simulink model "foc_fuzzy"  (R2025b)
settings: Solver=VariableStepAuto  StartTime=0.0  StopTime=3  RelTol=1e-3
libraries: slpidlib x2, spsSVPWMGenerator2LevelLib x1, spsdq0toAlphaBetaZeroLib x1, spsPermanentMagnetSynchronousMachineLib x1, spsDCVoltageSourceLib x1, spsThreePhaseVIMeasurementLib x1, spsUniversalBridgeLib x1, fuzblock x1, spsAlphaBetaZerotodq0Lib x1, spsabctoAlphaBetaZeroLib x1, sps_lib x1
settings Model: Creator=DELL  LastModifiedBy=DELL
settings DataIOCC: SaveState=on  SignalLogging=off  DSMLogging=off  ReturnWorkspaceOutputs=off

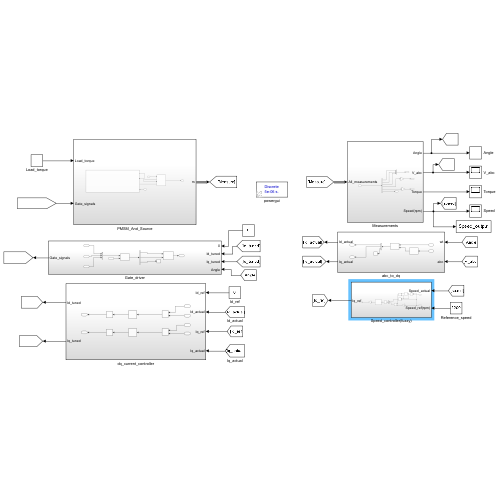
[thumbnail: Simulink's stored preview of the top-level diagram]
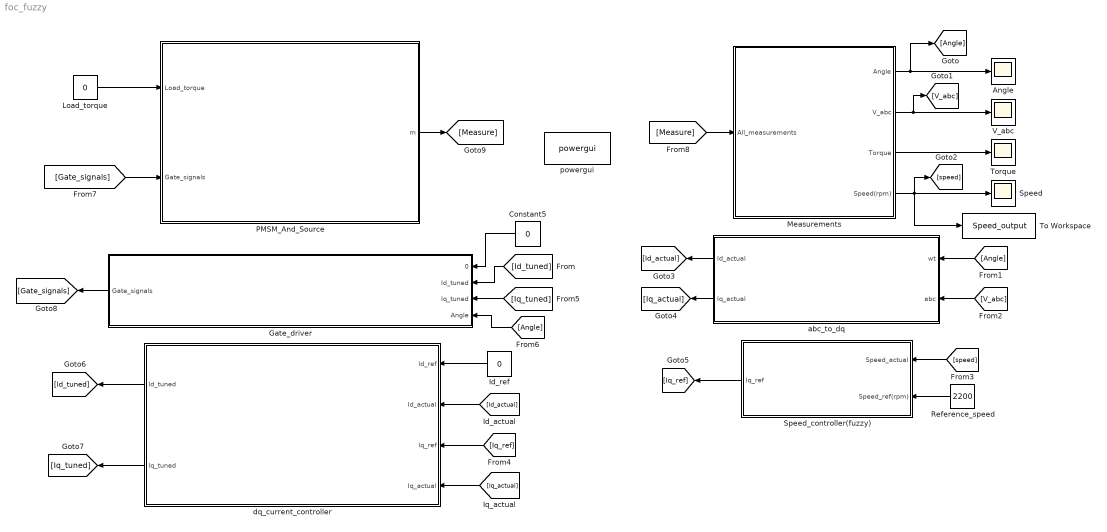
== system foc_fuzzy ==
  Angle : Scope
  Constant5 : Constant  Value=0
  Gate_driver : Subsystem
  Id_ref : Constant  Value=0
  Load_torque : Constant  Value=0
  Measurements : Subsystem
  PMSM_And_Source : Subsystem
  Reference_speed : Constant  Value=2200
  Speed : Scope
      settings: ActiveDisplayYMinimum=-270.85965206876136  ActiveDisplayYMaximum=2437.7368686188529  DataLoggingVariableName=ScopeData3
  Speed_controller(fuzzy) : Subsystem
      settings: PortSchema="{\"entries\":[{\"content\":{\"sides\":[{\"content\":{\"connectorIds\":[\"Out1\"]},\"type\":\"ConnectorPlacement.EquallySpacedRectSide\",\"uuid\":\"a1cd0f4b-38ea-419f-afc2-39e9bc7b0de2\"},{\"content\":{\"connectorIds\":[\"In1\",\"In2\"],\"side\":\"RIGHT\"},\"type\":\"ConnectorPlacement.EquallySpacedRectSide\",\"uuid\":\"efef469d-788b-4725-983f-524fe539f85d\"},{\"content\":{\"side\":\"TOP\"},\"type\":\"ConnectorPlacement.EquallySpacedRectSide\",\"uuid\":\"0e401ee3-352a-4969-a305-667f2f0ad6e7\"}]},\"type\":\"ConnectorPlacement.EquallySpacedConnector\",\"uuid\":\"94f18982-1906-49e5-aac5-92abf80968c3\"}],\"packageUris\":[\"http://schema.mathworks.com/mf0/Connector/R2020b\"],\"version\":\"1.0\"}"
  To Workspace : ToWorkspace  VariableName=Speed_output  SampleTime=-1
  Torque : Scope
      settings: DataLoggingVariableName=ScopeData2
  V_abc : Scope
  abc_to_dq : Subsystem
      settings: PortSchema="{\"entries\":[{\"content\":{\"sides\":[{\"content\":{\"connectorIds\":[\"Out1\",\"Out2\"]},\"type\":\"ConnectorPlacement.EquallySpacedRectSide\",\"uuid\":\"7ac698e7-d270-4bd0-8d73-3bcbd5b3bd28\"},{\"content\":{\"connectorIds\":[\"In1\",\"In2\"],\"side\":\"RIGHT\"},\"type\":\"ConnectorPlacement.EquallySpacedRectSide\",\"uuid\":\"e26e1610-01d9-4f07-bf5c-31b1329ae751\"},{\"content\":{\"side\":\"TOP\"},\"type\":\"ConnectorPlacement.EquallySpacedRectSide\",\"uuid\":\"585fc40b-a7d1-43b5-ab48-882fc2ec0db2\"}]},\"type\":\"ConnectorPlacement.EquallySpacedConnector\",\"uuid\":\"4680cdbc-79eb-4a7f-9529-209119af11d2\"}],\"packageUris\":[\"http://schema.mathworks.com/mf0/Connector/R2020b\"],\"version\":\"1.0\"}"
  dq_current_controller : Subsystem
      settings: PortSchema="{\"entries\":[{\"content\":{\"sides\":[{\"content\":{\"connectorIds\":[\"Out1\",\"Out2\"]},\"type\":\"ConnectorPlacement.EquallySpacedRectSide\",\"uuid\":\"85abe6a4-f46d-437d-9d29-ea06215c210d\"},{\"content\":{\"connectorIds\":[\"In1\",\"In2\",\"In3\",\"In4\"],\"side\":\"RIGHT\"},\"type\":\"ConnectorPlacement.EquallySpacedRectSide\",\"uuid\":\"dede3f64-84eb-4a1d-a083-0a7c4f3ca0cd\"},{\"content\":{\"side\":\"TOP\"},\"type\":\"ConnectorPlacement.EquallySpacedRectSide\",\"uuid\":\"b0cb4f54-dbd0-4970-9888-3ed028a2486f\"}]},\"type\":\"ConnectorPlacement.EquallySpacedConnector\",\"uuid\":\"91272fe0-95ae-4ab4-bc55-5dc81673f5f4\"}],\"packageUris\":[\"http://schema.mathworks.com/mf0/Connector/R2020b\"],\"version\":\"1.0\"}"
  powergui : sps_lib/powergui  Priority=1  SimulationMode=Discrete  SampleTime=5e-6  frequency=60  Iterations=50  frequencyindice=0  Pbase=100e6  ErrMax=1e-4  UnitsV=kV  UnitsW=MW  buscounter=0  FunctionMessages=off  echomessages=off  EnableUseOfTLC=off  CurrentSourceSwitches=off  DisableSnubberDevices=off  DisableRonSwitches=off  DisableVfSwitches=off  DisplayEquations=off  AutomaticDiscreteSolvers=off  SolverType=Tustin/Backward Euler (TBE)  Interpol=off  ExternalGateDelay=off  methode=off  Ts=100  x0status=blocks  SPID=on  SwTol=0  HookPort=off  NonlinearTolerance=1e-4  nMaxIteration=100  ContinueOnMaxIteration=off  RestoreLinks=warning  ResistiveCurrentMeasurement=off  Frange=[0:2:500]  Ylog=off  Xlog=on  ShowGrid=off  save=off  variable=ZData  structure=0  ZoomFFT=off  StartTime=0.0  cycles=1  DisplayStyle=1  fundamental=60  FreqAxis=off  MaxFrequency=1000  frequencyindicesteady=1  RmsSteady=1  display=off
  wires:
  Measurements/1(Angle) -> [Angle], Angle/1
  Measurements/2(V_abc) -> V_abc/1, [V_abc]
  Measurements/4(Speed(rpm)) -> To Workspace/1, Speed/1, [speed]
  Measurements/3(Torque) -> Torque/1
  [speed] -> Speed_controller(fuzzy)/1(Speed_actual)
  [Angle] -> abc_to_dq/1(wt)
  [V_abc] -> abc_to_dq/2(abc)
  abc_to_dq/1(Id_actual) -> [Id_actual]
  abc_to_dq/2(Iq_actual) -> [Iq_actual]
  Speed_controller(fuzzy)/1(Iq_ref) -> [Iq_ref]
  Id_ref/1 -> dq_current_controller/1(Id_ref)
  [Id_actual] -> dq_current_controller/2(Id_actual)
  [Iq_ref] -> dq_current_controller/3(Iq_ref)
  [Iq_actual] -> dq_current_controller/4(Iq_actual)
  Constant5/1 -> Gate_driver/1(0)
  dq_current_controller/2(Iq_tuned) -> [Iq_tuned]
  dq_current_controller/1(Id_tuned) -> [Id_tuned]
  [Id_tuned] -> Gate_driver/2(Id_tuned)
  [Iq_tuned] -> Gate_driver/3(Iq_tuned)
  [Angle] -> Gate_driver/4(Angle)
  Gate_driver/1(Gate_signals) -> [Gate_signals]
  [Gate_signals] -> PMSM_And_Source/2(Gate_signals)
  PMSM_And_Source/1(m) -> [Measure]
  [Measure] -> Measurements/1(All_measurements)
  Load_torque/1 -> PMSM_And_Source/1(Load_torque)
  Reference_speed/1 -> Speed_controller(fuzzy)/2(Speed_ref(rpm))

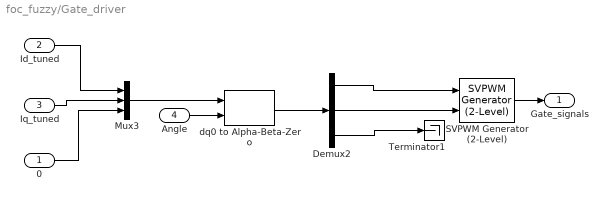
== system foc_fuzzy/Gate_driver ==
  0 : Inport
  Id_tuned : Inport  Port=2
  Iq_tuned : Inport  Port=3
  Angle : Inport  Port=4
  Demux2 : Demux  Outputs=3
  Mux3 : Mux  Inputs=3
  SVPWM Generator (2-Level) : spsSVPWMGenerator2LevelLib/SVPWM Generator (2-Level)  InputType=alpha-beta components  SwitchingPattern=Pattern #1  Fc=5000  ParUref=[0.8 -30 50]  Ts=0
  Terminator1 : Terminator
  dq0 to Alpha-Beta-Zero : spsdq0toAlphaBetaZeroLib/dq0 to Alpha-Beta-Zero  Alignment=90 degrees behind phase A axis
  Gate_signals : Outport
  wires:
  SVPWM Generator (2-Level)/1 -> Gate_signals/1
  Demux2/1 -> SVPWM Generator (2-Level)/1
  Demux2/2 -> SVPWM Generator (2-Level)/2
  Angle/1 -> dq0 to Alpha-Beta-Zero/2
  Demux2/3 -> Terminator1/1
  dq0 to Alpha-Beta-Zero/1 -> Demux2/1
  Mux3/1 -> dq0 to Alpha-Beta-Zero/1
  0/1 -> Mux3/3
  Id_tuned/1 -> Mux3/1
  Iq_tuned/1 -> Mux3/2

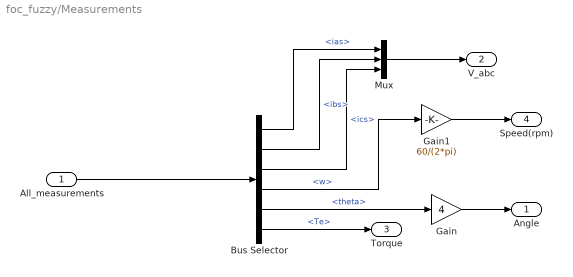
== system foc_fuzzy/Measurements ==
  All_measurements : Inport
  Bus Selector : BusSelector  OutputSignals=ias,ibs,ics,w,theta,Te
  Gain : Gain  Gain=4
  Gain1 : Gain  Gain=60/(2*pi)
  Mux : Mux  Inputs=3
  Angle : Outport
  V_abc : Outport  Port=2
  Torque : Outport  Port=3  VectorParamsAs1DForOutWhenUnconnected=off
  Speed(rpm) : Outport  Port=4
  wires:
  Mux/1 -> V_abc/1
  Gain1/1 -> Speed(rpm)/1
  Bus Selector/4 -> Gain1/1  "<w>"
  Bus Selector/6 -> Torque/1  "<Te>"
  Bus Selector/5 -> Gain/1  "<theta>"
  Bus Selector/3 -> Mux/3  "<ics>"
  Gain/1 -> Angle/1
  Bus Selector/1 -> Mux/1  "<ias>"
  Bus Selector/2 -> Mux/2  "<ibs>"
  All_measurements/1 -> Bus Selector/1

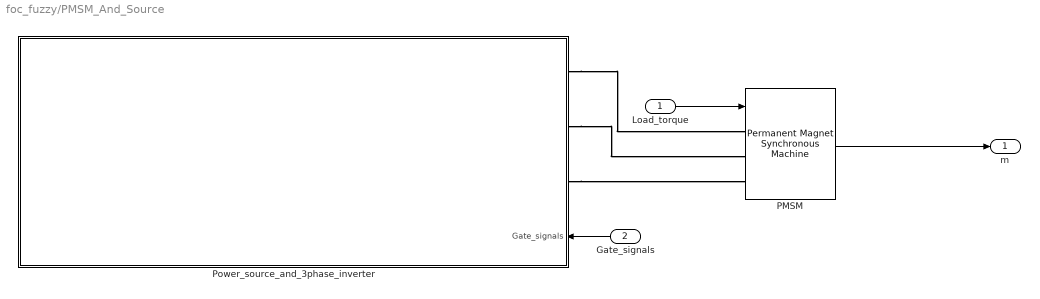
== system foc_fuzzy/PMSM_And_Source ==
  Load_torque : Inport
  Gate_signals : Inport  Port=2
  PMSM : spsPermanentMagnetSynchronousMachineLib/Permanent Magnet Synchronous Machine  NbPhases=3  FluxDistribution=Sinusoidal  RotorType=Round  MechanicalLoad=Torque Tm  PresetModel=No  ShowDetailedParameters=on  MeasurementBus=on  Resistance=0.0485  Inductance=8.5e-3  dqInductances=[8.5e-3,8.5e-3]  La=0.000395  MachineConstant=Flux linkage established by magnets (V.s)  Flux=0.1194  VoltageCst=86.6271  TorqueCst=0.7164  Flat=120  Mechanical=[0.0027 0.0004924 4 0]  PolePairs=4  InitialConditions=[0,0, 0,0]  InitialConditions5ph=[0 0 0 0 0 0]  RefAngle=90 degrees behind phase A axis (modified Park)  IterativeDiscreteModel=Trapezoidal non iterative  TsBlock=-1  TsPowergui=0
  Power_source_and_3phase_inverter : Subsystem
      settings: PortSchema="{\"entries\":[{\"content\":{\"sides\":[{\"content\":{},\"type\":\"ConnectorPlacement.EquallySpacedRectSide\",\"uuid\":\"19b577a6-4f33-43ed-8a86-594f3e9d4e9f\"},{\"content\":{\"connectorIds\":[\"RConn1\",\"RConn2\",\"RConn3\",\"In1\"],\"side\":\"RIGHT\"},\"type\":\"ConnectorPlacement.EquallySpacedRectSide\",\"uuid\":\"0fadcd66-7a34-426d-a0ad-26c1e66a9b65\"},{\"content\":{\"side\":\"TOP\"},\"type\":\"ConnectorPlacement.EquallySpacedRectSide\",\"uuid\":\"dc426c0c-5235-4165-aef9-5d4f6cb705db\"},{\"content\":{\"side\":\"BOTTOM\"},\"type\":\"ConnectorPlacement.EquallySpacedRectSide\",\"uuid\":\"557160c3-f5ce-40a2-884a-1c35634b9c5c\"}]},\"type\":\"ConnectorPlacement.EquallySpacedConnector\",\"uuid\":\"a5e7b64c-fcd0-4e18-89e2-e2da7a2362d3\"}],\"packageUris\":[\"http://schema.mathworks.com/mf0/Connector/R2020b\"],\"version\":\"1.0\"}"
  m : Outport
  wires:
  Load_torque/1 -> PMSM/1
  PMSM/1 -> m/1
  Gate_signals/1 -> Power_source_and_3phase_inverter/1(Gate_signals)
  connections:
  Power_source_and_3phase_inverter/RConn1 -- PMSM/LConn1
  Power_source_and_3phase_inverter/RConn2 -- PMSM/LConn2
  Power_source_and_3phase_inverter/RConn3 -- PMSM/LConn3

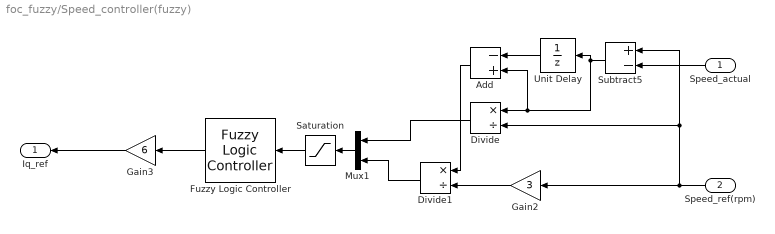
== system foc_fuzzy/Speed_controller(fuzzy) ==
  Speed_actual : Inport
  Speed_ref(rpm) : Inport  Port=2
  Add : Sum  Inputs=-+
  Divide : Product  Inputs=*/
  Divide1 : Product  Inputs=*/
  Fuzzy Logic Controller : fuzblock/Fuzzy Logic  Controller  FIS='fuzzy_controller.fis'  OutputSampleNumber=101  DataType=double  UseLookupTable=off  NumBreakpoints=2  FuzzifiedInputs=off  RuleFiringStrengths=off  RuleOutputs=off  AggregatedOutputs=off  SimulateUsing=Interpreted execution  OutOfRangeInputValueMessage=warning  NoRuleFiredMessage=warning  EmptyOutputFuzzySetMessage=warning
  Gain2 : Gain  Gain=3
  Gain3 : Gain  Gain=6
  Mux1 : Mux  Inputs=2
  Saturation : Saturate  UpperLimit=1  LowerLimit=-1
  Subtract5 : Sum  Inputs=+-
  Unit Delay : UnitDelay  SampleTime=-1  HasFrameUpgradeWarning=on
  Iq_ref : Outport
  wires:
  Unit Delay/1 -> Add/1
  Gain2/1 -> Divide1/2
  Speed_ref(rpm)/1 -> Divide/2, Subtract5/1, Gain2/1
  Subtract5/1 -> Add/2, Divide/1, Unit Delay/1
  Divide1/1 -> Mux1/2
  Divide/1 -> Mux1/1
  Mux1/1 -> Saturation/1
  Saturation/1 -> Fuzzy Logic Controller/1
  Fuzzy Logic Controller/1 -> Gain3/1
  Add/1 -> Divide1/1
  Speed_actual/1 -> Subtract5/2
  Gain3/1 -> Iq_ref/1

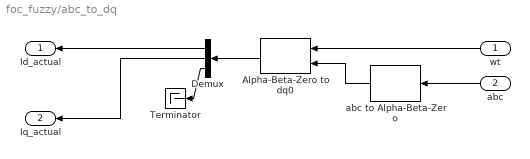
== system foc_fuzzy/abc_to_dq ==
  wt : Inport
  abc : Inport  Port=2
  Alpha-Beta-Zero to dq0 : spsAlphaBetaZerotodq0Lib/Alpha-Beta-Zero to dq0  Alignment=90 degrees behind phase A axis
  Demux : Demux  Outputs=3
  Terminator : Terminator
  abc to Alpha-Beta-Zero : spsabctoAlphaBetaZeroLib/abc to Alpha-Beta-Zero
  Id_actual : Outport
  Iq_actual : Outport  Port=2
  wires:
  Demux/3 -> Terminator/1
  Alpha-Beta-Zero to dq0/1 -> Demux/1
  abc/1 -> abc to Alpha-Beta-Zero/1
  abc to Alpha-Beta-Zero/1 -> Alpha-Beta-Zero to dq0/1
  Demux/2 -> Iq_actual/1
  wt/1 -> Alpha-Beta-Zero to dq0/2
  Demux/1 -> Id_actual/1

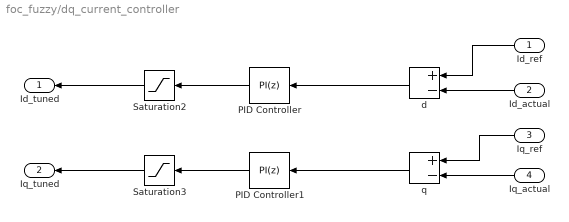
== system foc_fuzzy/dq_current_controller ==
  Id_ref : Inport
  Id_actual : Inport  Port=2
  Iq_ref : Inport  Port=3
  Iq_actual : Inport  Port=4
  PID Controller : slpidlib/PID Controller  Controller=PI  Form=Parallel  TimeDomain=Discrete-time  UseExternalTs=off  SampleTime=5e-06  IntegratorMethod=Forward Euler  FilterMethod=Forward Euler  ControllerParametersSource=internal  P=0.3  I=2  UseKiTs=off  D=0  UseExternalDerivativeSource=off  N=100  UseFilter=on  TunerSelectOption=Transfer Function Based (PID Tuner App)  InitialConditionSource=internal  InitialConditionForIntegrator=0  InitialConditionForFilter=0  DifferentiatorICPrevScaledInput=0  ExternalReset=none  TrackingMode=off  Kt=1  LimitOutput=off  SatLimitsSource=internal  UpperSaturationLimit=50  LowerSaturationLimit=-50  LinearizeAsGain=on  AntiWindupMode=none  Kb=1  LimitIntegrator=off  UpperIntegratorSaturationLimit=350/(1.732)  LowerIntegratorSaturationLimit=-350/(1.732)  POutMin=[]  POutMax=[]  IOutMin=[]  IOutMax=[]  DOutMin=[]  DOutMax=[]  NOutMin=[]  NOutMax=[]  SumOutMin=[]  SumOutMax=[]  SaturationOutMin=[]  SaturationOutMax=[]  PParamMin=[]  PParamMax=[]  IParamMin=[]  IParamMax=[]  DParamMin=[]  DParamMax=[]  NParamMin=[]  NParamMax=[]  KbParamMin=[]  KbParamMax=[]  KtParamMin=[]  KtParamMax=[]  KbOutMin=[]  KbOutMax=[]  KtOutMin=[]  KtOutMax=[]  IntegratorOutMin=[]  IntegratorOutMax=[]  FilterOutMin=[]  FilterOutMax=[]  SumI1OutMin=[]  SumI1OutMax=[]  SumI2OutMin=[]  SumI2OutMax=[]  SumI3OutMin=[]  SumI3OutMax=[]  SumI4OutMin=[]  SumI4OutMax=[]  SumDOutMin=[]  SumDOutMax=[]  DifferentiatorOutMin=[]  DifferentiatorOutMax=[]  FilterDiffOutCoefMin=[]  FilterDiffOutCoefMax=[]  ReciprocalOutMin=[]  ReciprocalOutMax=[]  SumDenOutMin=[]  SumDenOutMax=[]  SumNumOutMin=[]  SumNumOutMax=[]  DivideOutMin=[]  DivideOutMax=[]  UdiffTsProdOutMin=[]  UdiffTsProdOutMax=[]  NTsProdOutMin=[]  NTsProdOutMax=[]  UintegralTsProdOutMin=[]  UintegralTsProdOutMax=[]  UngainTsProdOutMin=[]  UngainTsProdOutMax=[]  ClampingZeroOutDataTypeStr=Inherit: Inherit via back propagation  ClampingZeroOutMin=[]  ClampingZeroOutMax=[]  FilterDenConstantOutDataTypeStr=Inherit: Inherit via back propagation  FilterDenConstantOutMin=[]  FilterDenConstantOutMax=[]  PCopyOutDataTypeStr=Inherit: Inherit via back propagation  PCopyOutMin=[]  PCopyOutMax=[]  NCopyOutDataTypeStr=Inherit: Inherit via back propagation  NCopyOutMin=[]  NCopyOutMax=[]  IntegratorContinuousStateAttributes=''  IntegratorStateMustResolveToSignalObject=off  IntegratorRTWStateStorageClass=Auto  FilterContinuousStateAttributes=''  FilterStateMustResolveToSignalObject=off  FilterRTWStateStorageClass=Auto  ParallelPVariant=InternalParameters  IdealPVariant=Disabled  IVariant=InternalParameters  DVariant=Disabled  IntegratorVariant=Discrete  SatVariant=Disabled  AWVariant=Passthrough  PCopyVariant=Disabled  TRVariant=Disabled  FdbkBlocksVariant=Forward  IdealPFdbkVariant=Disabled  SatFdbkVariant=Disabled  DerivativeFilterVariant=Disabled  NVariant=Disabled  NCopyVariant=Disabled_SignalSpec  FilterICVariant=Disabled  IntegratorICVariant=InternalICs  ExternalResetVariant=Disabled  TRSumVariant=Passthrough  SumFdbkVariant=Disabled  SumVariant=Sum_PI  TsampFilterVariant=InternalTs  TsampNgainVariant=Passthrough  TsampIntegralVariant=Disabled_SignalSpec  ExternalSaturationOutDataTypeStr=Inherit: Same as second input  DerivativeSourceVariant=Disabled  PreIntVariant=InternalPreInt
  PID Controller1 : slpidlib/PID Controller  Controller=PI  Form=Parallel  TimeDomain=Discrete-time  UseExternalTs=off  SampleTime=5e-06  IntegratorMethod=Forward Euler  FilterMethod=Forward Euler  ControllerParametersSource=internal  P=0.3  I=2  UseKiTs=off  D=0  UseExternalDerivativeSource=off  N=100  UseFilter=on  TunerSelectOption=Transfer Function Based (PID Tuner App)  InitialConditionSource=internal  InitialConditionForIntegrator=0  InitialConditionForFilter=0  DifferentiatorICPrevScaledInput=0  ExternalReset=none  TrackingMode=off  Kt=1  LimitOutput=off  SatLimitsSource=internal  UpperSaturationLimit=350/(1.732)  LowerSaturationLimit=-350/(1.732)  LinearizeAsGain=on  AntiWindupMode=none  Kb=1  LimitIntegrator=off  UpperIntegratorSaturationLimit=350/(1.732)  LowerIntegratorSaturationLimit=-350/(1.732)  POutMin=[]  POutMax=[]  IOutMin=[]  IOutMax=[]  DOutMin=[]  DOutMax=[]  NOutMin=[]  NOutMax=[]  SumOutMin=[]  SumOutMax=[]  SaturationOutMin=[]  SaturationOutMax=[]  PParamMin=[]  PParamMax=[]  IParamMin=[]  IParamMax=[]  DParamMin=[]  DParamMax=[]  NParamMin=[]  NParamMax=[]  KbParamMin=[]  KbParamMax=[]  KtParamMin=[]  KtParamMax=[]  KbOutMin=[]  KbOutMax=[]  KtOutMin=[]  KtOutMax=[]  IntegratorOutMin=[]  IntegratorOutMax=[]  FilterOutMin=[]  FilterOutMax=[]  SumI1OutMin=[]  SumI1OutMax=[]  SumI2OutMin=[]  SumI2OutMax=[]  SumI3OutMin=[]  SumI3OutMax=[]  SumI4OutMin=[]  SumI4OutMax=[]  SumDOutMin=[]  SumDOutMax=[]  DifferentiatorOutMin=[]  DifferentiatorOutMax=[]  FilterDiffOutCoefMin=[]  FilterDiffOutCoefMax=[]  ReciprocalOutMin=[]  ReciprocalOutMax=[]  SumDenOutMin=[]  SumDenOutMax=[]  SumNumOutMin=[]  SumNumOutMax=[]  DivideOutMin=[]  DivideOutMax=[]  UdiffTsProdOutMin=[]  UdiffTsProdOutMax=[]  NTsProdOutMin=[]  NTsProdOutMax=[]  UintegralTsProdOutMin=[]  UintegralTsProdOutMax=[]  UngainTsProdOutMin=[]  UngainTsProdOutMax=[]  ClampingZeroOutDataTypeStr=Inherit: Inherit via back propagation  ClampingZeroOutMin=[]  ClampingZeroOutMax=[]  FilterDenConstantOutDataTypeStr=Inherit: Inherit via back propagation  FilterDenConstantOutMin=[]  FilterDenConstantOutMax=[]  PCopyOutDataTypeStr=Inherit: Inherit via back propagation  PCopyOutMin=[]  PCopyOutMax=[]  NCopyOutDataTypeStr=Inherit: Inherit via back propagation  NCopyOutMin=[]  NCopyOutMax=[]  IntegratorContinuousStateAttributes=''  IntegratorStateMustResolveToSignalObject=off  IntegratorRTWStateStorageClass=Auto  FilterContinuousStateAttributes=''  FilterStateMustResolveToSignalObject=off  FilterRTWStateStorageClass=Auto  ParallelPVariant=InternalParameters  IdealPVariant=Disabled  IVariant=InternalParameters  DVariant=Disabled  IntegratorVariant=Discrete  SatVariant=Disabled  AWVariant=Passthrough  PCopyVariant=Disabled  TRVariant=Disabled  FdbkBlocksVariant=Forward  IdealPFdbkVariant=Disabled  SatFdbkVariant=Disabled  DerivativeFilterVariant=Disabled  NVariant=Disabled  NCopyVariant=Disabled_SignalSpec  FilterICVariant=Disabled  IntegratorICVariant=InternalICs  ExternalResetVariant=Disabled  TRSumVariant=Passthrough  SumFdbkVariant=Disabled  SumVariant=Sum_PI  TsampFilterVariant=InternalTs  TsampNgainVariant=Passthrough  TsampIntegralVariant=Disabled_SignalSpec  ExternalSaturationOutDataTypeStr=Inherit: Same as second input  DerivativeSourceVariant=Disabled  PreIntVariant=InternalPreInt
  Saturation2 : Saturate  UpperLimit=350/1.732  LowerLimit=-350/1.732
  Saturation3 : Saturate  UpperLimit=350/1.732  LowerLimit=-350/1.732
  d : Sum  Inputs=+-
  q : Sum  Inputs=+-
  Id_tuned : Outport
  Iq_tuned : Outport  Port=2
  wires:
  q/1 -> PID Controller1/1
  Saturation2/1 -> Id_tuned/1
  Saturation3/1 -> Iq_tuned/1
  Iq_ref/1 -> q/1
  PID Controller/1 -> Saturation2/1
  PID Controller1/1 -> Saturation3/1
  d/1 -> PID Controller/1
  Id_actual/1 -> d/2
  Id_ref/1 -> d/1
  Iq_actual/1 -> q/2

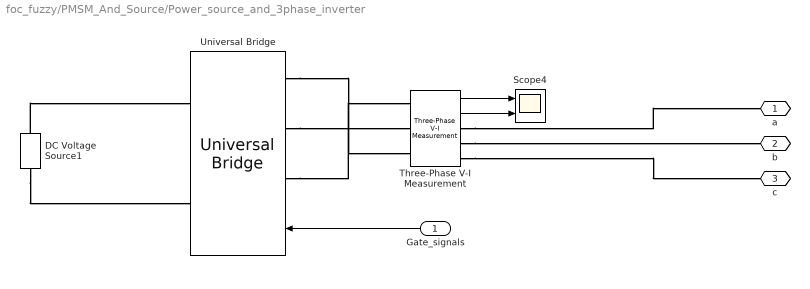
== system foc_fuzzy/PMSM_And_Source/Power_source_and_3phase_inverter ==
  Gate_signals : Inport
  DC Voltage Source1 : spsDCVoltageSourceLib/DC Voltage Source  Amplitude=350  Measurements=None
  Scope4 : Scope  NumInputPorts=2
      settings: ActiveDisplayYMinimum=-437.52115139486625  ActiveDisplayYMaximum=437.51926285940863  DataLoggingVariableName=ScopeData8
  Three-Phase V-I Measurement : spsThreePhaseVIMeasurementLib/Three-Phase V-I Measurement  VoltageMeasurement=phase-to-phase  SetLabelV=off  LabelV=Vabc  Vpu=off  VpuLL=off  CurrentMeasurement=yes  SetLabelI=off  LabelI=Iabc  Ipu=off  Pbase=100e6  Vbase=500e3  OutputType=Complex  PhasorSimulation=off  PSBequivalent=0
  Universal Bridge : spsUniversalBridgeLib/Universal Bridge  Arms=3  SnubberResistance=1e5  SnubberCapacitance=inf  Device=IGBT / Diodes  Ron=1e-3  Lon=0  ForwardVoltages="[  0  0  ]"  ForwardVoltage=0  GTOparameters=[ 10e-6 , 20e-6 ]  IGBTparameters=[ 1e-6 , 2e-6 ]  Measurements=None  Measurements_2=None  converterType=Rectifier
  a : PMIOPort  Side=Right
  b : PMIOPort  Port=2  Side=Right
  c : PMIOPort  Port=3  Side=Right
  wires:
  Three-Phase V-I Measurement/2 -> Scope4/2
  Three-Phase V-I Measurement/1 -> Scope4/1
  Gate_signals/1 -> Universal Bridge/1
  connections:
  Universal Bridge/LConn2 -- Three-Phase V-I Measurement/LConn2
  DC Voltage Source1/LConn1 -- Universal Bridge/RConn2
  Three-Phase V-I Measurement/RConn3 -- c/RConn1
  Universal Bridge/LConn1 -- Three-Phase V-I Measurement/LConn1
  Universal Bridge/LConn3 -- Three-Phase V-I Measurement/LConn3
  DC Voltage Source1/RConn1 -- Universal Bridge/RConn1
  Three-Phase V-I Measurement/RConn1 -- a/RConn1
  Three-Phase V-I Measurement/RConn2 -- b/RConn1
